simulink model "Memory_Buffer"  (R2024b)
settings: Solver=VariableStepAuto  StartTime=0.0  StopTime=10.0  RelTol=1e-3
settings Model: Creator=HP  LastModifiedBy=HP

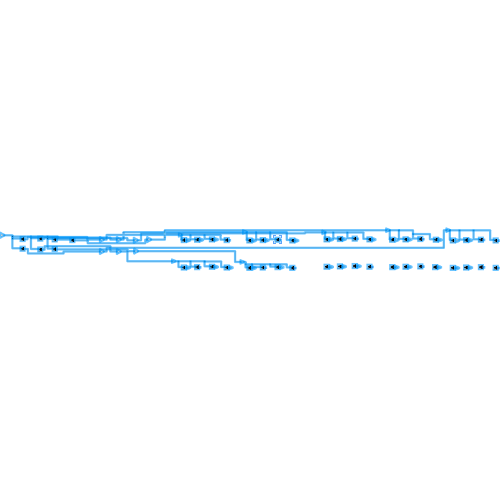
[thumbnail: Simulink's stored preview of the top-level diagram]
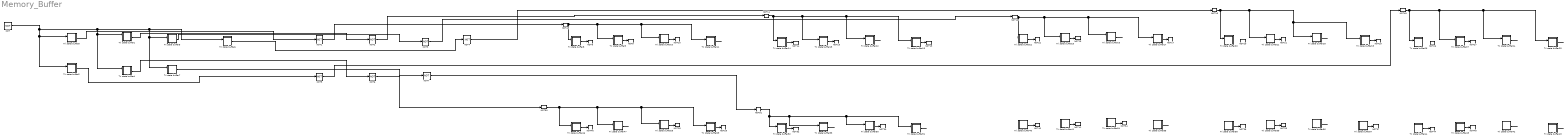
== system Memory_Buffer ==
  NOT{,1..17,19..23,26..30,32,34,37..41,44..46,48..51} (42 alike) : Logic  Operator=NOT  IconShape=distinctive  AllPortsSameDT=off  OutDataTypeStr=boolean
  Tri state buffer1 : Subsystem
      mask Display:
      | % Draw the triangle
      | patch([1 0 1], [0 0.5 1], [0 0 0])  % Left-pointing triangle
  Tri state buffer10 : Subsystem
      mask Display:
      | % Draw the triangle
      | patch([1 0 1], [0 0.5 1], [0 0 0])  % Left-pointing triangle
  Tri state buffer11 : Subsystem
      mask Display:
      | % Draw the triangle
      | patch([1 0 1], [0 0.5 1], [0 0 0])  % Left-pointing triangle
  Tri state buffer12 : Subsystem
      mask Display:
      | % Draw the triangle
      | patch([1 0 1], [0 0.5 1], [0 0 0])  % Left-pointing triangle
  Tri state buffer13 : Subsystem
      mask Display:
      | % Draw the triangle
      | patch([1 0 1], [0 0.5 1], [0 0 0])  % Left-pointing triangle
  Tri state buffer14 : Subsystem
      mask Display:
      | % Draw the triangle
      | patch([1 0 1], [0 0.5 1], [0 0 0])  % Left-pointing triangle
  Tri state buffer15 : Subsystem
      mask Display:
      | % Draw the triangle
      | patch([1 0 1], [0 0.5 1], [0 0 0])  % Left-pointing triangle
  Tri state buffer16 : Subsystem
      mask Display:
      | % Draw the triangle
      | patch([1 0 1], [0 0.5 1], [0 0 0])  % Left-pointing triangle
  Tri state buffer17 : Subsystem
      mask Display:
      | % Draw the triangle
      | patch([1 0 1], [0 0.5 1], [0 0 0])  % Left-pointing triangle
  Tri state buffer18 : Subsystem
      mask Display:
      | % Draw the triangle
      | patch([1 0 1], [0 0.5 1], [0 0 0])  % Left-pointing triangle
  Tri state buffer19 : Subsystem
      mask Display:
      | % Draw the triangle
      | patch([1 0 1], [0 0.5 1], [0 0 0])  % Left-pointing triangle
  Tri state buffer2 : Subsystem
      mask Display:
      | % Draw the triangle
      | patch([1 0 1], [0 0.5 1], [0 0 0])  % Left-pointing triangle
  Tri state buffer20 : Subsystem
      mask Display:
      | % Draw the triangle
      | patch([1 0 1], [0 0.5 1], [0 0 0])  % Left-pointing triangle
  Tri state buffer21 : Subsystem
      mask Display:
      | % Draw the triangle
      | patch([1 0 1], [0 0.5 1], [0 0 0])  % Left-pointing triangle
  Tri state buffer22 : Subsystem
      mask Display:
      | % Draw the triangle
      | patch([1 0 1], [0 0.5 1], [0 0 0])  % Left-pointing triangle
  Tri state buffer23 : Subsystem
      mask Display:
      | % Draw the triangle
      | patch([1 0 1], [0 0.5 1], [0 0 0])  % Left-pointing triangle
  Tri state buffer24 : Subsystem
      mask Display:
      | % Draw the triangle
      | patch([1 0 1], [0 0.5 1], [0 0 0])  % Left-pointing triangle
  Tri state buffer25 : Subsystem
      mask Display:
      | % Draw the triangle
      | patch([1 0 1], [0 0.5 1], [0 0 0])  % Left-pointing triangle
  Tri state buffer26 : Subsystem
      mask Display:
      | % Draw the triangle
      | patch([1 0 1], [0 0.5 1], [0 0 0])  % Left-pointing triangle
  Tri state buffer27 : Subsystem
      mask Display:
      | % Draw the triangle
      | patch([1 0 1], [0 0.5 1], [0 0 0])  % Left-pointing triangle
  Tri state buffer28 : Subsystem
      mask Display:
      | % Draw the triangle
      | patch([1 0 1], [0 0.5 1], [0 0 0])  % Left-pointing triangle
  Tri state buffer29 : Subsystem
      mask Display:
      | % Draw the triangle
      | patch([1 0 1], [0 0.5 1], [0 0 0])  % Left-pointing triangle
  Tri state buffer3 : Subsystem
      mask Display:
      | % Draw the triangle
      | patch([1 0 1], [0 0.5 1], [0 0 0])  % Left-pointing triangle
  Tri state buffer30 : Subsystem
      mask Display:
      | % Draw the triangle
      | patch([1 0 1], [0 0.5 1], [0 0 0])  % Left-pointing triangle
  Tri state buffer31 : Subsystem
      mask Display:
      | % Draw the triangle
      | patch([1 0 1], [0 0.5 1], [0 0 0])  % Left-pointing triangle
  Tri state buffer32 : Subsystem
      mask Display:
      | % Draw the triangle
      | patch([1 0 1], [0 0.5 1], [0 0 0])  % Left-pointing triangle
  Tri state buffer33 : Subsystem
      mask Display:
      | % Draw the triangle
      | patch([1 0 1], [0 0.5 1], [0 0 0])  % Left-pointing triangle
  Tri state buffer34 : Subsystem
      mask Display:
      | % Draw the triangle
      | patch([1 0 1], [0 0.5 1], [0 0 0])  % Left-pointing triangle
  Tri state buffer35 : Subsystem
      mask Display:
      | % Draw the triangle
      | patch([1 0 1], [0 0.5 1], [0 0 0])  % Left-pointing triangle
  Tri state buffer36 : Subsystem
      mask Display:
      | % Draw the triangle
      | patch([1 0 1], [0 0.5 1], [0 0 0])  % Left-pointing triangle
  Tri state buffer37 : Subsystem
      mask Display:
      | % Draw the triangle
      | patch([1 0 1], [0 0.5 1], [0 0 0])  % Left-pointing triangle
  Tri state buffer38 : Subsystem
      mask Display:
      | % Draw the triangle
      | patch([1 0 1], [0 0.5 1], [0 0 0])  % Left-pointing triangle
  Tri state buffer39 : Subsystem
      mask Display:
      | % Draw the triangle
      | patch([1 0 1], [0 0.5 1], [0 0 0])  % Left-pointing triangle
  Tri state buffer4 : Subsystem
      mask Display:
      | % Draw the triangle
      | patch([1 0 1], [0 0.5 1], [0 0 0])  % Left-pointing triangle
  Tri state buffer40 : Subsystem
      mask Display:
      | % Draw the triangle
      | patch([1 0 1], [0 0.5 1], [0 0 0])  % Left-pointing triangle
  Tri state buffer41 : Subsystem
      mask Display:
      | % Draw the triangle
      | patch([1 0 1], [0 0.5 1], [0 0 0])  % Left-pointing triangle
  Tri state buffer42 : Subsystem
      mask Display:
      | % Draw the triangle
      | patch([1 0 1], [0 0.5 1], [0 0 0])  % Left-pointing triangle
  Tri state buffer43 : Subsystem
      mask Display:
      | % Draw the triangle
      | patch([1 0 1], [0 0.5 1], [0 0 0])  % Left-pointing triangle
  Tri state buffer44 : Subsystem
      mask Display:
      | % Draw the triangle
      | patch([1 0 1], [0 0.5 1], [0 0 0])  % Left-pointing triangle
  Tri state buffer45 : Subsystem
      mask Display:
      | % Draw the triangle
      | patch([1 0 1], [0 0.5 1], [0 0 0])  % Left-pointing triangle
  Tri state buffer46 : Subsystem
      mask Display:
      | % Draw the triangle
      | patch([1 0 1], [0 0.5 1], [0 0 0])  % Left-pointing triangle
  Tri state buffer47 : Subsystem
      mask Display:
      | % Draw the triangle
      | patch([1 0 1], [0 0.5 1], [0 0 0])  % Left-pointing triangle
  Tri state buffer5 : Subsystem
      mask Display:
      | % Draw the triangle
      | patch([1 0 1], [0 0.5 1], [0 0 0])  % Left-pointing triangle
  Tri state buffer6 : Subsystem
      mask Display:
      | % Draw the triangle
      | patch([1 0 1], [0 0.5 1], [0 0 0])  % Left-pointing triangle
  Tri state buffer7 : Subsystem
      mask Display:
      | % Draw the triangle
      | patch([1 0 1], [0 0.5 1], [0 0 0])  % Left-pointing triangle
  Tri state buffer8 : Subsystem
      mask Display:
      | % Draw the triangle
      | patch([1 0 1], [0 0.5 1], [0 0 0])  % Left-pointing triangle
  Tri state buffer9 : Subsystem
      mask Display:
      | % Draw the triangle
      | patch([1 0 1], [0 0.5 1], [0 0 0])  % Left-pointing triangle
  wires:
  NOT/1 -> Tri state buffer6/1(In1), Tri state buffer7/1(In1), Tri state buffer5/1(In1), Tri state buffer4/1(In1), Tri state buffer1/1(In1), Tri state buffer2/1(In1), Tri state buffer3/1(In1)
  Tri state buffer3/1(Out1) -> NOT1/1
  Tri state buffer1/1(Out1) -> NOT2/1
  Tri state buffer5/1(Out1) -> NOT3/1
  Tri state buffer6/1(Out1) -> NOT4/1
  Tri state buffer2/1(Out1) -> NOT5/1
  Tri state buffer4/1(Out1) -> NOT6/1
  Tri state buffer7/1(Out1) -> NOT7/1
  Tri state buffer9/1(Out1) -> NOT9/1
  Tri state buffer10/1(Out1) -> NOT10/1
  Tri state buffer11/1(Out1) -> ?
  Tri state buffer13/1(Out1) -> NOT13/1
  Tri state buffer12/1(Out1) -> ?
  Tri state buffer15/1(Out1) -> NOT15/1
  Tri state buffer21/1(Out1) -> NOT21/1
  Tri state buffer18/1(Out1) -> ?
  Tri state buffer19/1(Out1) -> NOT19/1
  Tri state buffer17/1(Out1) -> NOT17/1
  Tri state buffer16/1(Out1) -> ?
  Tri state buffer23/1(Out1) -> NOT23/1
  Tri state buffer25/1(Out1) -> ?
  Tri state buffer24/1(Out1) -> ?
  Tri state buffer27/1(Out1) -> NOT27/1
  Tri state buffer45/1(Out1) -> NOT45/1
  Tri state buffer42/1(Out1) -> ?
  Tri state buffer43/1(Out1) -> ?
  Tri state buffer41/1(Out1) -> NOT41/1
  Tri state buffer34/1(Out1) -> NOT34/1
  Tri state buffer35/1(Out1) -> ?
  Tri state buffer37/1(Out1) -> NOT37/1
  Tri state buffer36/1(Out1) -> ?
  Tri state buffer39/1(Out1) -> NOT39/1
  Tri state buffer33/1(Out1) -> ?
  Tri state buffer30/1(Out1) -> NOT30/1
  Tri state buffer31/1(Out1) -> ?
  Tri state buffer29/1(Out1) -> NOT29/1
  Tri state buffer28/1(Out1) -> NOT28/1
  Tri state buffer47/1(Out1) -> ?
  NOT1/1 -> NOT48/1
  NOT48/1 -> Tri state buffer11/1(In1), Tri state buffer10/1(In1), Tri state buffer9/1(In1), Tri state buffer8/1(In1)
  NOT2/1 -> NOT11/1
  NOT11/1 -> Tri state buffer13/1(In1), Tri state buffer12/1(In1), Tri state buffer15/1(In1), Tri state buffer14/1(In1)
  NOT3/1 -> NOT12/1
  NOT12/1 -> Tri state buffer17/1(In1), Tri state buffer16/1(In1), Tri state buffer23/1(In1), Tri state buffer22/1(In1)
  Tri state buffer22/1(Out1) -> NOT22/1
  NOT4/1 -> NOT16/1
  NOT16/1 -> Tri state buffer19/1(In1), Tri state buffer18/1(In1), Tri state buffer21/1(In1), Tri state buffer20/1(In1)
  NOT5/1 -> NOT49/1
  NOT49/1 -> Tri state buffer25/1(In1), Tri state buffer24/1(In1), Tri state buffer27/1(In1), Tri state buffer26/1(In1)
  NOT6/1 -> NOT50/1
  NOT50/1 -> Tri state buffer29/1(In1), Tri state buffer28/1(In1), Tri state buffer47/1(In1), Tri state buffer46/1(In1)
  NOT7/1 -> NOT51/1
  NOT51/1 -> Tri state buffer31/1(In1), Tri state buffer30/1(In1), Tri state buffer33/1(In1), Tri state buffer32/1(In1)
  Tri state buffer46/1(Out1) -> NOT46/1
  Tri state buffer8/1(Out1) -> NOT8/1
  Tri state buffer14/1(Out1) -> NOT14/1
  Tri state buffer32/1(Out1) -> NOT32/1
  Tri state buffer40/1(Out1) -> NOT40/1
  Tri state buffer38/1(Out1) -> NOT38/1
  Tri state buffer44/1(Out1) -> NOT44/1

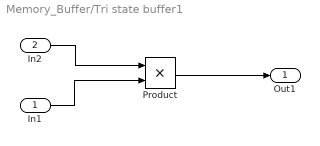
== system Memory_Buffer/Tri state buffer1 ==
  In1 : Inport
  In2 : Inport  Port=2
  Product : Product
  Out1 : Outport
  wires:
  In1/1 -> Product/2
  In2/1 -> Product/1
  Product/1 -> Out1/1

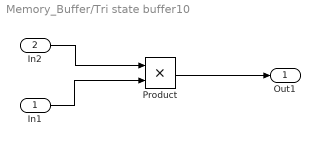
== system Memory_Buffer/Tri state buffer10 ==
  In1 : Inport
  In2 : Inport  Port=2
  Product : Product
  Out1 : Outport
  wires:
  Product/1 -> Out1/1
  In2/1 -> Product/1
  In1/1 -> Product/2

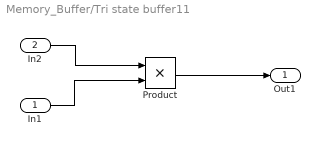
== system Memory_Buffer/Tri state buffer11 ==
  In1 : Inport
  In2 : Inport  Port=2
  Product : Product
  Out1 : Outport
  wires:
  In1/1 -> Product/2
  In2/1 -> Product/1
  Product/1 -> Out1/1

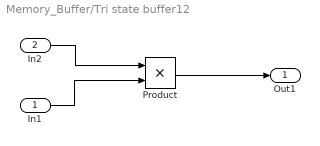
== system Memory_Buffer/Tri state buffer12 ==
  In1 : Inport
  In2 : Inport  Port=2
  Product : Product
  Out1 : Outport
  wires:
  In1/1 -> Product/2
  In2/1 -> Product/1
  Product/1 -> Out1/1

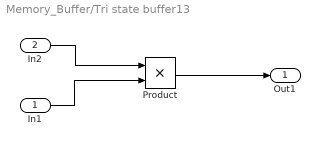
== system Memory_Buffer/Tri state buffer13 ==
  In1 : Inport
  In2 : Inport  Port=2
  Product : Product
  Out1 : Outport
  wires:
  Product/1 -> Out1/1
  In2/1 -> Product/1
  In1/1 -> Product/2

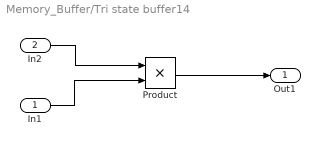
== system Memory_Buffer/Tri state buffer14 ==
  In1 : Inport
  In2 : Inport  Port=2
  Product : Product
  Out1 : Outport
  wires:
  In1/1 -> Product/2
  In2/1 -> Product/1
  Product/1 -> Out1/1

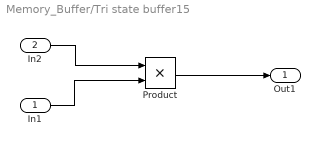
== system Memory_Buffer/Tri state buffer15 ==
  In1 : Inport
  In2 : Inport  Port=2
  Product : Product
  Out1 : Outport
  wires:
  Product/1 -> Out1/1
  In2/1 -> Product/1
  In1/1 -> Product/2

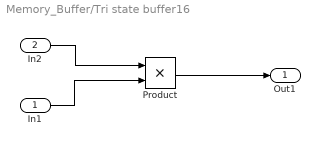
== system Memory_Buffer/Tri state buffer16 ==
  In1 : Inport
  In2 : Inport  Port=2
  Product : Product
  Out1 : Outport
  wires:
  In1/1 -> Product/2
  In2/1 -> Product/1
  Product/1 -> Out1/1

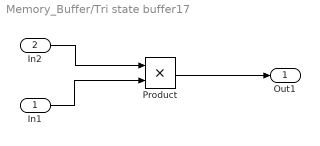
== system Memory_Buffer/Tri state buffer17 ==
  In1 : Inport
  In2 : Inport  Port=2
  Product : Product
  Out1 : Outport
  wires:
  Product/1 -> Out1/1
  In2/1 -> Product/1
  In1/1 -> Product/2

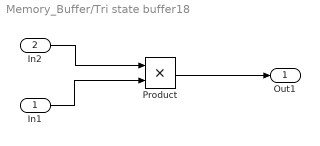
== system Memory_Buffer/Tri state buffer18 ==
  In1 : Inport
  In2 : Inport  Port=2
  Product : Product
  Out1 : Outport
  wires:
  Product/1 -> Out1/1
  In2/1 -> Product/1
  In1/1 -> Product/2

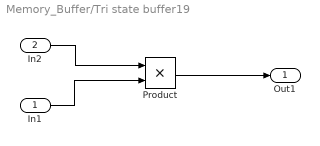
== system Memory_Buffer/Tri state buffer19 ==
  In1 : Inport
  In2 : Inport  Port=2
  Product : Product
  Out1 : Outport
  wires:
  In1/1 -> Product/2
  In2/1 -> Product/1
  Product/1 -> Out1/1

== system Memory_Buffer/Tri state buffer2 ==
  In1 : Inport
  In2 : Inport  Port=2
  Product : Product
  Out1 : Outport
  wires:
  Product/1 -> Out1/1
  In2/1 -> Product/1
  In1/1 -> Product/2

== system Memory_Buffer/Tri state buffer20 ==
  In1 : Inport
  In2 : Inport  Port=2
  Product : Product
  Out1 : Outport
  wires:
  Product/1 -> Out1/1
  In2/1 -> Product/1
  In1/1 -> Product/2

== system Memory_Buffer/Tri state buffer21 ==
  In1 : Inport
  In2 : Inport  Port=2
  Product : Product
  Out1 : Outport
  wires:
  In1/1 -> Product/2
  In2/1 -> Product/1
  Product/1 -> Out1/1

== system Memory_Buffer/Tri state buffer22 ==
  In1 : Inport
  In2 : Inport  Port=2
  Product : Product
  Out1 : Outport
  wires:
  In1/1 -> Product/2
  In2/1 -> Product/1
  Product/1 -> Out1/1

== system Memory_Buffer/Tri state buffer23 ==
  In1 : Inport
  In2 : Inport  Port=2
  Product : Product
  Out1 : Outport
  wires:
  Product/1 -> Out1/1
  In2/1 -> Product/1
  In1/1 -> Product/2

== system Memory_Buffer/Tri state buffer24 ==
  In1 : Inport
  In2 : Inport  Port=2
  Product : Product
  Out1 : Outport
  wires:
  In1/1 -> Product/2
  In2/1 -> Product/1
  Product/1 -> Out1/1

== system Memory_Buffer/Tri state buffer25 ==
  In1 : Inport
  In2 : Inport  Port=2
  Product : Product
  Out1 : Outport
  wires:
  Product/1 -> Out1/1
  In2/1 -> Product/1
  In1/1 -> Product/2

== system Memory_Buffer/Tri state buffer26 ==
  In1 : Inport
  In2 : Inport  Port=2
  Product : Product
  Out1 : Outport
  wires:
  In1/1 -> Product/2
  In2/1 -> Product/1
  Product/1 -> Out1/1

== system Memory_Buffer/Tri state buffer27 ==
  In1 : Inport
  In2 : Inport  Port=2
  Product : Product
  Out1 : Outport
  wires:
  Product/1 -> Out1/1
  In2/1 -> Product/1
  In1/1 -> Product/2

== system Memory_Buffer/Tri state buffer28 ==
  In1 : Inport
  In2 : Inport  Port=2
  Product : Product
  Out1 : Outport
  wires:
  In1/1 -> Product/2
  In2/1 -> Product/1
  Product/1 -> Out1/1

== system Memory_Buffer/Tri state buffer29 ==
  In1 : Inport
  In2 : Inport  Port=2
  Product : Product
  Out1 : Outport
  wires:
  Product/1 -> Out1/1
  In2/1 -> Product/1
  In1/1 -> Product/2

== system Memory_Buffer/Tri state buffer3 ==
  In1 : Inport
  In2 : Inport  Port=2
  Product : Product
  Out1 : Outport
  wires:
  Product/1 -> Out1/1
  In2/1 -> Product/1
  In1/1 -> Product/2

== system Memory_Buffer/Tri state buffer30 ==
  In1 : Inport
  In2 : Inport  Port=2
  Product : Product
  Out1 : Outport
  wires:
  Product/1 -> Out1/1
  In2/1 -> Product/1
  In1/1 -> Product/2

== system Memory_Buffer/Tri state buffer31 ==
  In1 : Inport
  In2 : Inport  Port=2
  Product : Product
  Out1 : Outport
  wires:
  In1/1 -> Product/2
  In2/1 -> Product/1
  Product/1 -> Out1/1

== system Memory_Buffer/Tri state buffer32 ==
  In1 : Inport
  In2 : Inport  Port=2
  Product : Product
  Out1 : Outport
  wires:
  Product/1 -> Out1/1
  In2/1 -> Product/1
  In1/1 -> Product/2

== system Memory_Buffer/Tri state buffer33 ==
  In1 : Inport
  In2 : Inport  Port=2
  Product : Product
  Out1 : Outport
  wires:
  In1/1 -> Product/2
  In2/1 -> Product/1
  Product/1 -> Out1/1

== system Memory_Buffer/Tri state buffer34 ==
  In1 : Inport
  In2 : Inport  Port=2
  Product : Product
  Out1 : Outport
  wires:
  Product/1 -> Out1/1
  In2/1 -> Product/1
  In1/1 -> Product/2

== system Memory_Buffer/Tri state buffer35 ==
  In1 : Inport
  In2 : Inport  Port=2
  Product : Product
  Out1 : Outport
  wires:
  In1/1 -> Product/2
  In2/1 -> Product/1
  Product/1 -> Out1/1

== system Memory_Buffer/Tri state buffer36 ==
  In1 : Inport
  In2 : Inport  Port=2
  Product : Product
  Out1 : Outport
  wires:
  In1/1 -> Product/2
  In2/1 -> Product/1
  Product/1 -> Out1/1

== system Memory_Buffer/Tri state buffer37 ==
  In1 : Inport
  In2 : Inport  Port=2
  Product : Product
  Out1 : Outport
  wires:
  Product/1 -> Out1/1
  In2/1 -> Product/1
  In1/1 -> Product/2

== system Memory_Buffer/Tri state buffer38 ==
  In1 : Inport
  In2 : Inport  Port=2
  Product : Product
  Out1 : Outport
  wires:
  In1/1 -> Product/2
  In2/1 -> Product/1
  Product/1 -> Out1/1

== system Memory_Buffer/Tri state buffer39 ==
  In1 : Inport
  In2 : Inport  Port=2
  Product : Product
  Out1 : Outport
  wires:
  Product/1 -> Out1/1
  In2/1 -> Product/1
  In1/1 -> Product/2

== system Memory_Buffer/Tri state buffer4 ==
  In1 : Inport
  In2 : Inport  Port=2
  Product : Product
  Out1 : Outport
  wires:
  In1/1 -> Product/2
  In2/1 -> Product/1
  Product/1 -> Out1/1

== system Memory_Buffer/Tri state buffer40 ==
  In1 : Inport
  In2 : Inport  Port=2
  Product : Product
  Out1 : Outport
  wires:
  Product/1 -> Out1/1
  In2/1 -> Product/1
  In1/1 -> Product/2

== system Memory_Buffer/Tri state buffer41 ==
  In1 : Inport
  In2 : Inport  Port=2
  Product : Product
  Out1 : Outport
  wires:
  In1/1 -> Product/2
  In2/1 -> Product/1
  Product/1 -> Out1/1

== system Memory_Buffer/Tri state buffer42 ==
  In1 : Inport
  In2 : Inport  Port=2
  Product : Product
  Out1 : Outport
  wires:
  Product/1 -> Out1/1
  In2/1 -> Product/1
  In1/1 -> Product/2

== system Memory_Buffer/Tri state buffer43 ==
  In1 : Inport
  In2 : Inport  Port=2
  Product : Product
  Out1 : Outport
  wires:
  In1/1 -> Product/2
  In2/1 -> Product/1
  Product/1 -> Out1/1

== system Memory_Buffer/Tri state buffer44 ==
  In1 : Inport
  In2 : Inport  Port=2
  Product : Product
  Out1 : Outport
  wires:
  Product/1 -> Out1/1
  In2/1 -> Product/1
  In1/1 -> Product/2

== system Memory_Buffer/Tri state buffer45 ==
  In1 : Inport
  In2 : Inport  Port=2
  Product : Product
  Out1 : Outport
  wires:
  In1/1 -> Product/2
  In2/1 -> Product/1
  Product/1 -> Out1/1

== system Memory_Buffer/Tri state buffer46 ==
  In1 : Inport
  In2 : Inport  Port=2
  Product : Product
  Out1 : Outport
  wires:
  In1/1 -> Product/2
  In2/1 -> Product/1
  Product/1 -> Out1/1

== system Memory_Buffer/Tri state buffer47 ==
  In1 : Inport
  In2 : Inport  Port=2
  Product : Product
  Out1 : Outport
  wires:
  Product/1 -> Out1/1
  In2/1 -> Product/1
  In1/1 -> Product/2

== system Memory_Buffer/Tri state buffer5 ==
  In1 : Inport
  In2 : Inport  Port=2
  Product : Product
  Out1 : Outport
  wires:
  Product/1 -> Out1/1
  In2/1 -> Product/1
  In1/1 -> Product/2

== system Memory_Buffer/Tri state buffer6 ==
  In1 : Inport
  In2 : Inport  Port=2
  Product : Product
  Out1 : Outport
  wires:
  In1/1 -> Product/2
  In2/1 -> Product/1
  Product/1 -> Out1/1

== system Memory_Buffer/Tri state buffer7 ==
  In1 : Inport
  In2 : Inport  Port=2
  Product : Product
  Out1 : Outport
  wires:
  Product/1 -> Out1/1
  In2/1 -> Product/1
  In1/1 -> Product/2

== system Memory_Buffer/Tri state buffer8 ==
  In1 : Inport
  In2 : Inport  Port=2
  Product : Product
  Out1 : Outport
  wires:
  Product/1 -> Out1/1
  In2/1 -> Product/1
  In1/1 -> Product/2

== system Memory_Buffer/Tri state buffer9 ==
  In1 : Inport
  In2 : Inport  Port=2
  Product : Product
  Out1 : Outport
  wires:
  In1/1 -> Product/2
  In2/1 -> Product/1
  Product/1 -> Out1/1
